simulink model "SPO10"  (R2018b)
settings: Solver=VariableStepAuto  StartTime=0.0  StopTime=0.1  RelTol=1e-3
undefined symbols (not defined in the file or in its folder): phased, physconst
libraries: powerlib_meascontrol x7, phasedwavlib x2, phasedtxrxlib x2, phasedenvlib x1, simulink x1
settings Model: SimulationMode=accelerator  Creator=matib  LastModifiedBy=matib
settings OptimizationCC: BooleanDataType=off

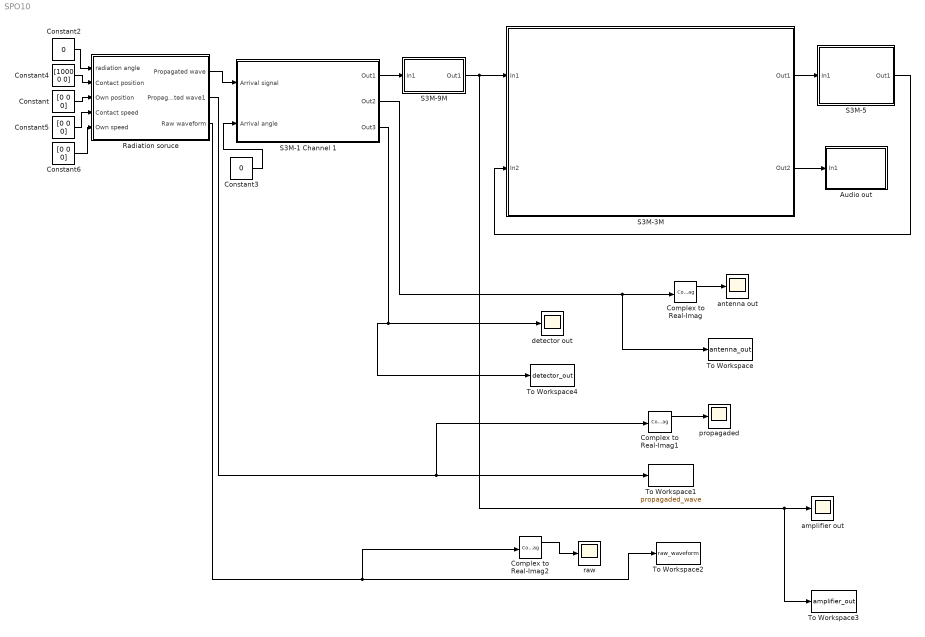
== system SPO10 ==
  Audio out : Subsystem
  Complex to Real-Imag : ComplexToRealImag
  Complex to Real-Imag1 : ComplexToRealImag
  Complex to Real-Imag2 : ComplexToRealImag
  Constant : Constant  Value=[0 0 0]
  Constant2 : Constant  Value=0
  Constant3 : Constant  Value=0
  Constant4 : Constant  Value=[1000 0 0]
  Constant5 : Constant  Value=[0 0 0]
  Constant6 : Constant  Value=[0 0 0]
  Radiation soruce : Subsystem
  S3M-1 Channel 1 : Subsystem
  S3M-3M : Subsystem
  S3M-5 : Subsystem
  S3M-9M : Subsystem
  To Workspace : ToWorkspace  VariableName=antenna_out  SaveFormat=Structure With Time  SampleTime=-1
  To Workspace1 : ToWorkspace  VariableName=propagaded_wave  SaveFormat=Structure With Time  SampleTime=-1
  To Workspace2 : ToWorkspace  VariableName=raw_waveform  SaveFormat=Structure With Time  SampleTime=-1
  To Workspace3 : ToWorkspace  VariableName=amplifier_out  SaveFormat=Structure With Time  SampleTime=-1
  To Workspace4 : ToWorkspace  VariableName=detector_out  SaveFormat=Structure With Time  SampleTime=-1
  amplifier out : Scope
  antenna out : Scope
  detector out : Scope
  propagaded : Scope
  raw : Scope
  wires:
  S3M-1 Channel 1/1(Out1) -> S3M-9M/1(In1)
  Radiation soruce/1(Propagated wave) -> S3M-1 Channel 1/1(Arrival signal)
  S3M-3M/2(Out2) -> Audio out/1(In1)
  S3M-5/1(Out1) -> S3M-3M/2(In2)
  Constant/1 -> Radiation soruce/3(Own position)
  Constant2/1 -> Radiation soruce/1(radiation angle)
  Constant3/1 -> S3M-1 Channel 1/2(Arrival angle)
  Constant4/1 -> Radiation soruce/2(Contact position)
  Constant5/1 -> Radiation soruce/4(Contact speed)
  Constant6/1 -> Radiation soruce/5(Own speed)
  S3M-1 Channel 1/2(Out2) -> To Workspace/1, Complex to Real-Imag/1
  Radiation soruce/2(Propagated wave1) -> Complex to Real-Imag1/1, To Workspace1/1
  Radiation soruce/3(Raw waveform) -> Complex to Real-Imag2/1, To Workspace2/1
  Complex to Real-Imag/1 -> antenna out/1
  Complex to Real-Imag1/1 -> propagaded/1
  Complex to Real-Imag2/1 -> raw/1
  S3M-9M/1(Out1) -> amplifier out/1, To Workspace3/1, S3M-3M/1(In1)
  S3M-1 Channel 1/3(Out3) -> To Workspace4/1, detector out/1
  S3M-3M/1(Out1) -> S3M-5/1(In1)

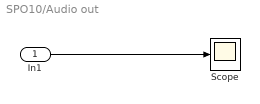
== system SPO10/Audio out ==
  In1 : Inport
  Scope : Scope
  wires:
  In1/1 -> Scope/1

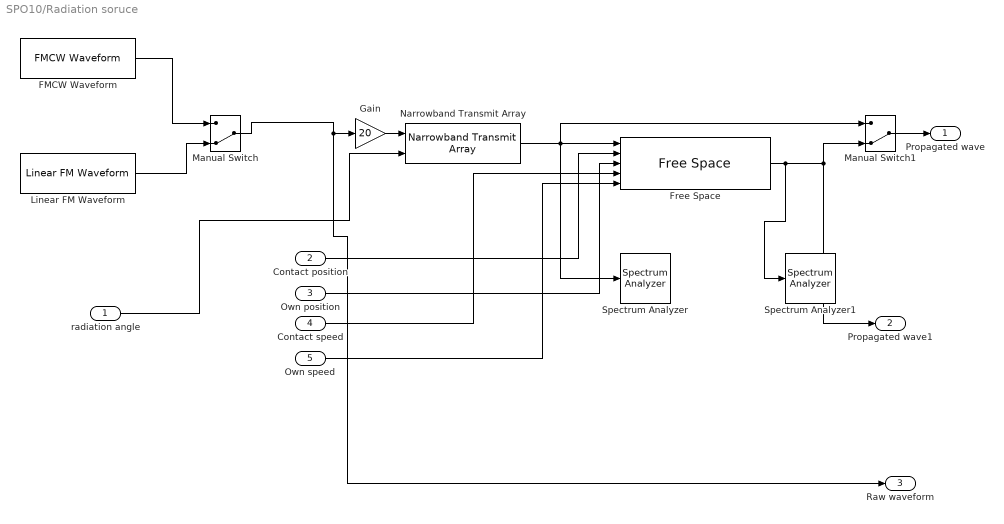
== system SPO10/Radiation soruce ==
  radiation angle : Inport
  Contact position : Inport  Port=2
  Own position : Inport  Port=3
  Contact speed : Inport  Port=4
  Own speed : Inport  Port=5
  FMCW Waveform : phasedwavlib/FMCW Waveform  SampleRate=1.5e7  SweepTime=1e-4  SweepBandwidth=6e6  SweepDirection=Triangle  SweepInterval=Positive  OutputFormat=Samples  NumSamples=100  NumSweeps=1  SimulateUsing=Interpreted execution
      settings: SourceProductName=Phased Array System Toolbox  SourceProductBaseCode=AR
  Free Space : phasedenvlib/Free Space  PropagationSpeed=physconst( 'LightSpeed' )  OperatingFrequency=3e8  TwoWayPropagation=off  SampleRateFromInputCheckbox=on  SampleRate=1e6  MaximumDistanceSource=Property  MaximumDistance=10e3  MaximumNumInputSamplesSource=Auto  MaximumNumInputSamples=1000  SimulateUsing=Interpreted execution
      settings: SourceProductName=Phased Array System Toolbox  SourceProductBaseCode=AR
  Gain : Gain  Gain=20
  Linear FM Waveform : phasedwavlib/Linear FM Waveform  SampleRate=1.5e7  DurationSpecification=Pulse width  PulseWidth=0.0001  DutyCycle=0.5  PRF=4e3  PRFSelectionInputPort=off  SimulationTimeSource=Derive from waveform parameters  SweepBandwidth=6e6  SweepDirection=Up  SweepInterval=Positive  Envelope=Rectangular  OutputFormat=Samples  NumSamples=100  NumPulses=1  PRFOutputPort=off  SimulateUsing=Interpreted execution
      settings: SourceProductName=Phased Array System Toolbox  SourceProductBaseCode=AR
  Manual Switch : ManualSwitch  CurrentSetting=0
  Manual Switch1 : ManualSwitch  CurrentSetting=0
  Narrowband Transmit Array : phasedtxrxlib/Narrowband Transmit Array  PropagationSpeed=physconst( 'LightSpeed' )  OperatingFrequency=3e8  CombineRadiatedSignals=on  SensorGainMeasure=dB  Polarization=None  WeightsInputPort=off  SimulateUsing=Interpreted execution  Sensor=phased.URA('Element',phased.IsotropicAntennaElement())
      settings: SourceProductName=Phased Array System Toolbox  SourceProductBaseCode=AR
  Spectrum Analyzer : SpectrumAnalyzer
  Spectrum Analyzer1 : SpectrumAnalyzer
  Propagated wave : Outport
  Propagated wave1 : Outport  Port=2
  Raw waveform : Outport  Port=3
  wires:
  Manual Switch/1 -> Raw waveform/1, Gain/1
  radiation angle/1 -> Narrowband Transmit Array/2
  Narrowband Transmit Array/1 -> Spectrum Analyzer/1, Manual Switch1/1, Free Space/1
  Free Space/1 -> Spectrum Analyzer1/1, Propagated wave1/1, Manual Switch1/2
  Contact position/1 -> Free Space/2
  Own position/1 -> Free Space/3
  Contact speed/1 -> Free Space/4
  Own speed/1 -> Free Space/5
  FMCW Waveform/1 -> Manual Switch/1
  Linear FM Waveform/1 -> Manual Switch/2
  Gain/1 -> Narrowband Transmit Array/1
  Manual Switch1/1 -> Propagated wave/1

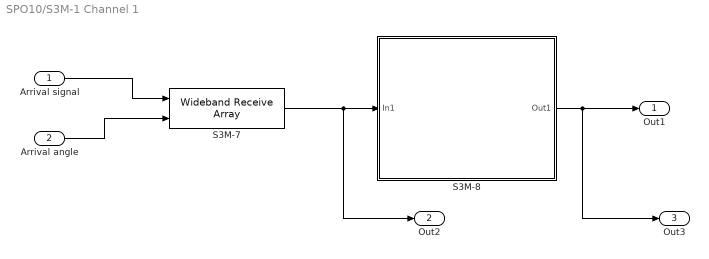
== system SPO10/S3M-1 Channel 1 ==
  Arrival signal : Inport
  Arrival angle : Inport  Port=2
  S3M-7 : phasedtxrxlib/Wideband Receive Array  PropagationSpeed=physconst( 'LightSpeed' )  SampleRateFromInputCheckbox=on  SampleRate=1e6  ModulatedInput=on  CarrierFrequency=8e9  NumSubbands=64  Wavefront=Plane  SensorGainMeasure=dB  Polarization=None  WeightsInputPort=off  SimulateUsing=Interpreted execution  Sensor=SZM7
      settings: SourceProductName=Phased Array System Toolbox  SourceProductBaseCode=AR
  S3M-8 : Subsystem
  Out1 : Outport
  Out2 : Outport  Port=2
  Out3 : Outport  Port=3
  wires:
  S3M-7/1 -> Out2/1, S3M-8/1(In1)
  Arrival signal/1 -> S3M-7/1
  Arrival angle/1 -> S3M-7/2
  S3M-8/1(Out1) -> Out1/1, Out3/1

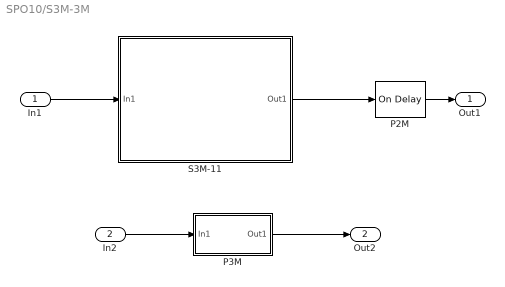
== system SPO10/S3M-3M ==
  In1 : Inport
  In2 : Inport  Port=2
  P2M : powerlib_meascontrol/Logic/On Delay  DelayType=On delay  delay=0.0001  ic=0  Ts=0
      settings: SourceProductName=Simscape Power Systems
  P3M : Subsystem
  S3M-11 : Subsystem
  Out1 : Outport
  Out2 : Outport  Port=2
  wires:
  In1/1 -> S3M-11/1(In1)
  S3M-11/1(Out1) -> P2M/1
  P2M/1 -> Out1/1
  P3M/1(Out1) -> Out2/1
  In2/1 -> P3M/1(In1)

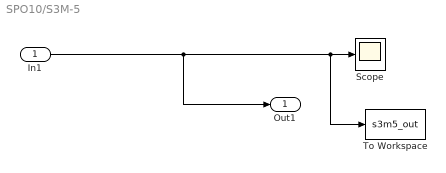
== system SPO10/S3M-5 ==
  In1 : Inport
  Scope : Scope
  To Workspace : ToWorkspace  VariableName=s3m5_out  SaveFormat=Timeseries  SampleTime=-1
  Out1 : Outport
  wires:
  In1/1 -> Out1/1, To Workspace/1, Scope/1

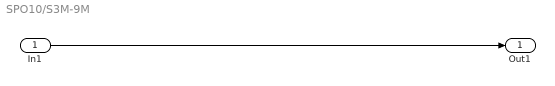
== system SPO10/S3M-9M ==
  In1 : Inport
  Out1 : Outport
  wires:
  In1/1 -> Out1/1

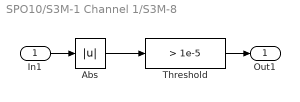
== system SPO10/S3M-1 Channel 1/S3M-8 ==
  In1 : Inport
  Abs : Abs
  Threshold : simulink/Logic and Bit Operations/Compare To Constant  relop=>  const=1e-5  OutDataTypeStr=boolean  ZeroCross=off
  Out1 : Outport
  wires:
  Threshold/1 -> Out1/1
  In1/1 -> Abs/1
  Abs/1 -> Threshold/1

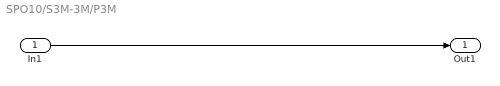
== system SPO10/S3M-3M/P3M ==
  In1 : Inport
  Out1 : Outport
  wires:
  In1/1 -> Out1/1

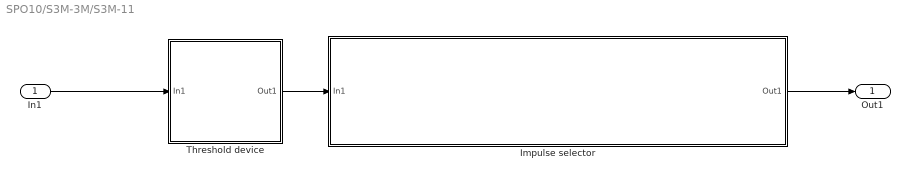
== system SPO10/S3M-3M/S3M-11 ==
  In1 : Inport
  Impulse selector : Subsystem
  "Threshold device " : Subsystem
  Out1 : Outport
  wires:
  In1/1 -> "Threshold device "/1(In1)
  "Threshold device "/1(Out1) -> Impulse selector/1(In1)
  Impulse selector/1(Out1) -> Out1/1

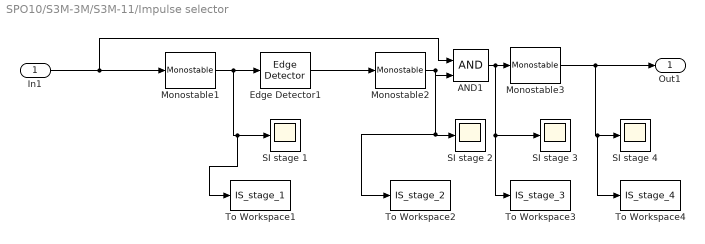
== system SPO10/S3M-3M/S3M-11/Impulse selector ==
  In1 : Inport
  AND1 : Logic  IconShape=distinctive  AllPortsSameDT=off  OutDataTypeStr=boolean
  Edge Detector1 : powerlib_meascontrol/Logic/Edge Detector  model=Falling  ic=0  Ts=0
      settings: SourceProductName=Simscape Power Systems  SourceProductBaseCode=PS
  Monostable1 : powerlib_meascontrol/Logic/Monostable  EdgeDetect=Rising  PulseDuration=4.05e-4  ic=0  Ts=0
      settings: SourceProductName=Simscape Power Systems  SourceProductBaseCode=PS
  Monostable2 : powerlib_meascontrol/Logic/Monostable  EdgeDetect=Rising  PulseDuration=7.9e-4  ic=0  Ts=0
      settings: SourceProductName=Simscape Power Systems  SourceProductBaseCode=PS
  Monostable3 : powerlib_meascontrol/Logic/Monostable  EdgeDetect=Rising  PulseDuration=0.08  ic=0  Ts=0
      settings: SourceProductName=Simscape Power Systems  SourceProductBaseCode=PS
  SI stage {1..4} (4 alike) : Scope
  To Workspace1 : ToWorkspace  VariableName=IS_stage_1  SaveFormat=Timeseries  SampleTime=-1
  To Workspace2 : ToWorkspace  VariableName=IS_stage_2  SaveFormat=Timeseries  SampleTime=-1
  To Workspace3 : ToWorkspace  VariableName=IS_stage_3  SaveFormat=Timeseries  SampleTime=-1
  To Workspace4 : ToWorkspace  VariableName=IS_stage_4  SaveFormat=Timeseries  SampleTime=-1
  Out1 : Outport
  wires:
  In1/1 -> AND1/1, Monostable1/1
  Monostable2/1 -> To Workspace2/1, SI stage 2/1, AND1/2
  Monostable1/1 -> To Workspace1/1, SI stage 1/1, Edge Detector1/1
  Monostable3/1 -> To Workspace4/1, SI stage 4/1, Out1/1
  Edge Detector1/1 -> Monostable2/1
  AND1/1 -> To Workspace3/1, SI stage 3/1, Monostable3/1

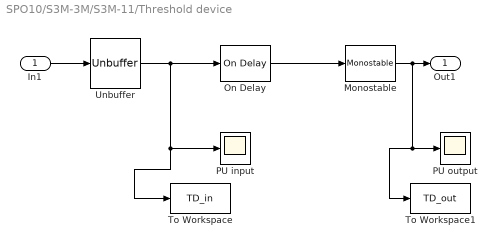
== system SPO10/S3M-3M/S3M-11/Threshold device  ==
  In1 : Inport
  Monostable : powerlib_meascontrol/Logic/Monostable  EdgeDetect=Rising  PulseDuration=20e-6  ic=0  Ts=0
      settings: SourceProductName=Simscape Power Systems  SourceProductBaseCode=PS
  On Delay : powerlib_meascontrol/Logic/On Delay  DelayType=On delay  delay=5e-6  ic=0  Ts=0
      settings: SourceProductName=Simscape Power Systems
  PU input : Scope
  PU output : Scope
  To Workspace : ToWorkspace  VariableName=TD_in  SaveFormat=Timeseries  SampleTime=-1
  To Workspace1 : ToWorkspace  VariableName=TD_out  SaveFormat=Timeseries  SampleTime=-1
  Unbuffer : Unbuffer
  Out1 : Outport
  wires:
  On Delay/1 -> Monostable/1
  In1/1 -> Unbuffer/1
  Unbuffer/1 -> To Workspace/1, PU input/1, On Delay/1
  Monostable/1 -> PU output/1, To Workspace1/1, Out1/1
